simulink model "EMK"  (R2022b)
settings: Solver=VariableStepAuto  StartTime=0.0  StopTime=10.0  RelTol=1e-3
settings Model: Creator=Noor Hakam  LastModifiedBy=Noor Hakam

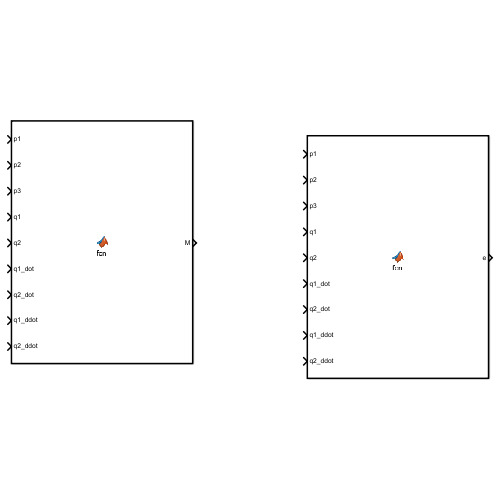
[thumbnail: Simulink's stored preview of the top-level diagram]
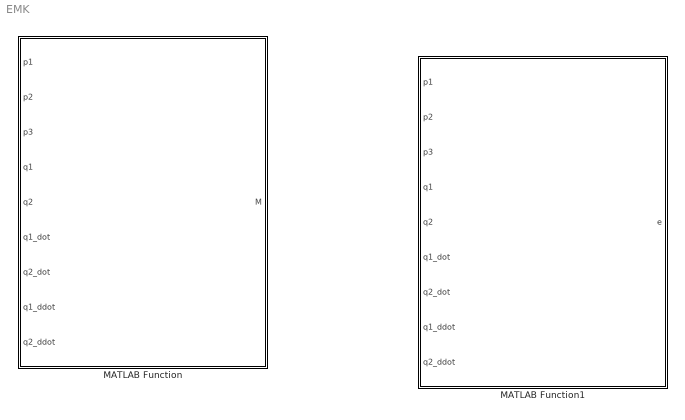
== system EMK ==
  MATLAB Function : MATLAB Function  TreatAsAtomicUnit=on
  MATLAB Function1 : MATLAB Function  TreatAsAtomicUnit=on

== matlab function EMK/MATLAB Function1 ==
  data: p1 input; e output; p2 input; p3 input; q1 input; q2 input; q1_dot input; q2_dot input; q1_ddot input; q2_ddot input
function e = fcn(p1, p2, p3, q1, q2, q1_dot, q2_dot, q1_ddot, q2_ddot)

y = u;

== matlab function EMK/MATLAB Function ==
  data: p1 input; M output; p2 input; p3 input; q1 input; q2 input; q1_dot input; q2_dot input; q1_ddot input; q2_ddot input
function M = fcn(p1, p2, p3, q1, q2, q1_dot, q2_dot, q1_ddot, q2_ddot)

y = u;
